simulink model "baseline_auto_parcel_loading_process"  (R2026a)
settings: Solver=VariableStepAuto  StopTime=500  MaxStep=0.05
libraries: sim3dlib x36
(part 5 of 5)

== matlab function baseline_auto_parcel_loading_process/MultiFloorUnloadPrepositionFunction ==
  data: mission_phase input size=[1 1]; unload_floor1_conv_cmd output size=[1 1]; vehicle_stopped input size=[1 1]; delivery_arrived input; target_index_f1 input size=[1 1]; found_f1 input size=[1 1]; target_id_f1 input size=[1 1]; target_index_f2 input size=[1 1]; found_f2 input size=[1 1]; target_id_f2 input size=[1 1]; target_index_f3 input size=[1 1]; found_f3 input size=[1 1]; target_id_f3 input size=[1 1]; unload_floor2_conv_cmd output size=[1 1]; unload_floor3_conv_cmd output size=[1 1]; sensor_count_f1 output size=[1 1]; sensor_count_f2 output size=[1 1]; sensor_count_f3 output size=[1 1]; target_on_belt4_f1 output size=[1 1]; target_on_belt4_f2 output size=[1 1]; target_on_belt4_f3 output size=[1 1]; preposition_active_f1 output size=[1 1]; preposition_active_f2 output size=[1 1]; preposition_active_f3 output size=[1 1]; unload_state_id_for_preposition input size=[1 1]; visual_shift_f1 output size=[1 1]; visual_shift_f2 output size=[1 1]; visual_shift_f3 output size=[1 1]
function [unload_floor1_conv_cmd, unload_floor2_conv_cmd, unload_floor3_conv_cmd, ...
          sensor_count_f1, sensor_count_f2, sensor_count_f3, ...
          target_on_belt4_f1, target_on_belt4_f2, target_on_belt4_f3, ...
          preposition_active_f1, preposition_active_f2, preposition_active_f3, ...
          visual_shift_f1, visual_shift_f2, visual_shift_f3] = ...
          MultiFloorUnloadPrepositionFunction( ...
          mission_phase, vehicle_stopped, delivery_arrived, ...
          target_index_f1, found_f1, target_id_f1, ...
          target_index_f2, found_f2, target_id_f2, ...
          target_index_f3, found_f3, target_id_f3, ...
          unload_state_id_for_preposition)
% MultiFloorUnloadPrepositionFunction
%
% 목적:
% - 배송 중 정차 시간에 각 층 컨베이어를 독립적으로 순환시켜
%   각 층의 하차 대상 1개씩을 Belt4 상단/플랫폼 앞 하차공간으로 미리 이동시킨다.
%
% 추가 목적:
% - 같은 층에 하차 대상이 여러 개 있을 때,
%   첫 번째 하차 후 다음 대상도 다시 하차공간으로 준비할 수 있게 한다.
%
% 이번 추가:
% - visual_shift_f1/f2/f3 출력
% - sensor_count는 정수 칸 이동량
% - visual_shift는 정수 칸 이동량 + 현재 카운트 사이의 진행률
%
% 핵심 규칙:
% - mission_phase == 1 일 때만 하차 준비 가능
% - vehicle_stopped == 1 일 때만 하차 준비 가능
% - 배송 중(delivery_arrived == 0)에는 정차 중이면 준비 가능
% - 배달 장소 도착 후(delivery_arrived == 1)에는 UnloadController가 IDLE일 때만 준비 가능
% - 실제 하차 중(unload_state_id 1~7)에는 준비 컨베이어 정지
% - 각 층 sensor_count는 독립적으로 관리
% - queue 자체는 회전시키지 않고, 표시용 sensor_count/visual_shift만 증가시킴
%
% 중요:
% - target_index = 1 이라고 해서 즉시 하차공간에 있다고 보지 않는다.
% - 실제 시스템의 카운팅은 "첫 번째 택배 통과 = count 1"이다.
% - 따라서 필요한 count는 target_index - 1 이 아니라 target_index 이다.

persistent count_f1 count_f2 count_f3
persistent step_f1 step_f2 step_f3
persistent done_f1 done_f2 done_f3
persistent prev_target_id_f1 prev_target_id_f2 prev_target_id_f3

if isempty(count_f1)
    count_f1 = 0;
    count_f2 = 0;
    count_f3 = 0;

    step_f1 = 0;
    step_f2 = 0;
    step_f3 = 0;

    done_f1 = 0;
    done_f2 = 0;
    done_f3 = 0;

    prev_target_id_f1 = 0;
    prev_target_id_f2 = 0;
    prev_target_id_f3 = 0;
end

% =========================
% 조정 파라미터
% =========================
% Sample time = 0.05 기준
% COUNT_INTERVAL = 20이면 약 1초마다 sensor_count가 1 증가
COUNT_INTERVAL = 60;

% =========================
% 기본 출력
% =========================
unload_floor1_conv_cmd = 0;
unload_floor2_conv_cmd = 0;
unload_floor3_conv_cmd = 0;

target_on_belt4_f1 = 0;
target_on_belt4_f2 = 0;
target_on_belt4_f3 = 0;

preposition_active_f1 = 0;
preposition_active_f2 = 0;
preposition_active_f3 = 0;

% =========================
% target 변경 감지 및 층별 카운터 리셋
% =========================
if target_id_f1 ~= prev_target_id_f1
    count_f1 = 0;
    step_f1 = 0;
    done_f1 = 0;
    prev_target_id_f1 = target_id_f1;
end

if target_id_f2 ~= prev_target_id_f2
    count_f2 = 0;
    step_f2 = 0;
    done_f2 = 0;
    prev_target_id_f2 = target_id_f2;
end

if target_id_f3 ~= prev_target_id_f3
    count_f3 = 0;
    step_f3 = 0;
    done_f3 = 0;
    prev_target_id_f3 = target_id_f3;
end

% target이 없으면 해당 층 준비 상태 리셋
if found_f1 < 0.5 || target_id_f1 <= 0
    count_f1 = 0;
    step_f1 = 0;
    done_f1 = 0;
end

if found_f2 < 0.5 || target_id_f2 <= 0
    count_f2 = 0;
    step_f2 = 0;
    done_f2 = 0;
end

if found_f3 < 0.5 || target_id_f3 <= 0
    count_f3 = 0;
    step_f3 = 0;
    done_f3 = 0;
end

% =========================
% 필요한 sensor count 계산
% =========================
need_f1 = target_index_f1;
need_f2 = target_index_f2;
need_f3 = target_index_f3;

if need_f1 < 0
    need_f1 = 0;
end

if need_f2 < 0
    need_f2 = 0;
end

if need_f3 < 0
    need_f3 = 0;
end

if found_f1 < 0.5 || target_id_f1 <= 0
    need_f1 = 0;
end

if found_f2 < 0.5 || target_id_f2 <= 0
    need_f2 = 0;
end

if found_f3 < 0.5 || target_id_f3 <= 0
    need_f3 = 0;
end

% =========================
% 준비 완료 판정
% =========================
if found_f1 > 0.5 && target_id_f1 > 0
    if count_f1 >= need_f1
        done_f1 = 1;
    end
end

if found_f2 > 0.5 && target_id_f2 > 0
    if count_f2 >= need_f2
        done_f2 = 1;
    end
end

if found_f3 > 0.5 && target_id_f3 > 0
    if count_f3 >= need_f3
        done_f3 = 1;
    end
end

% =========================
% 하차 준비 허용 조건
% =========================
% 배송 중:
%   delivery_arrived = 0
%   vehicle_stopped = 1
%   → 준비 가능
%
% 배달 장소 도착 후:
%   delivery_arrived = 1
%   unload_state_id_for_preposition = 0
%   → 실제 하차 중이 아닐 때만 다음 대상 준비 가능
%
% 실제 하차 중:
%   unload_state_id_for_preposition ~= 0
%   → 준비 컨베이어 정지
prep_allowed = 0;

if mission_phase == 1 && vehicle_stopped > 0.5

    if delivery_arrived <= 0.5
        prep_allowed = 1;

    else
        if unload_state_id_for_preposition <= 0.5
            prep_allowed = 1;
        else
            prep_allowed = 0;
        end
    end

end

% =========================
% 1층 준비
% =========================
if found_f1 > 0.5 && target_id_f1 > 0 && done_f1 < 0.5
    if prep_allowed > 0.5
        preposition_active_f1 = 1;
        unload_floor1_conv_cmd = 1;

        step_f1 = step_f1 + 1;

        if step_f1 >= COUNT_INTERVAL
            step_f1 = 0;
            count_f1 = count_f1 + 1;
        end
    end
end

% =========================
% 2층 준비
% =========================
if found_f2 > 0.5 && target_id_f2 > 0 && done_f2 < 0.5
    if prep_allowed > 0.5
        preposition_active_f2 = 1;
        unload_floor2_conv_cmd = 1;

        step_f2 = step_f2 + 1;

        if step_f2 >= COUNT_INTERVAL
            step_f2 = 0;
            count_f2 = count_f2 + 1;
        end
    end
end

% =========================
% 3층 준비
% =========================
if found_f3 > 0.5 && target_id_f3 > 0 && done_f3 < 0.5
    if prep_allowed > 0.5
        preposition_active_f3 = 1;
        unload_floor3_conv_cmd = 1;

        step_f3 = step_f3 + 1;

        if step_f3 >= COUNT_INTERVAL
            step_f3 = 0;
            count_f3 = count_f3 + 1;
        end
    end
end

% =========================
% 준비 완료 재판정
% =========================
if found_f1 > 0.5 && target_id_f1 > 0
    if count_f1 >= need_f1
        done_f1 = 1;
    end
end

if found_f2 > 0.5 && target_id_f2 > 0
    if count_f2 >= need_f2
        done_f2 = 1;
    end
end

if found_f3 > 0.5 && target_id_f3 > 0
    if count_f3 >= need_f3
        done_f3 = 1;
    end
end

% =========================
% 출력
% =========================
sensor_count_f1 = count_f1;
sensor_count_f2 = count_f2;
sensor_count_f3 = count_f3;

if done_f1 > 0.5 && found_f1 > 0.5 && target_id_f1 > 0
    target_on_belt4_f1 = 1;
else
    target_on_belt4_f1 = 0;
end

if done_f2 > 0.5 && found_f2 > 0.5 && target_id_f2 > 0
    target_on_belt4_f2 = 1;
else
    target_on_belt4_f2 = 0;
end

if done_f3 > 0.5 && found_f3 > 0.5 && target_id_f3 > 0
    target_on_belt4_f3 = 1;
else
    target_on_belt4_f3 = 0;
end

% =========================
% 연속 이동 시각화용 출력
% =========================
% done 상태가 아니고, 실제로 준비 active 중일 때는
% count + step/COUNT_INTERVAL 값을 내보낸다.
%
% done 상태에서는 step이 남아 있어도 정수 count 위치로 고정한다.
if done_f1 < 0.5 && preposition_active_f1 > 0.5
    visual_shift_f1 = count_f1 + step_f1 / COUNT_INTERVAL;
else
    visual_shift_f1 = count_f1;
end

if done_f2 < 0.5 && preposition_active_f2 > 0.5
    visual_shift_f2 = count_f2 + step_f2 / COUNT_INTERVAL;
else
    visual_shift_f2 = count_f2;
end

if done_f3 < 0.5 && preposition_active_f3 > 0.5
    visual_shift_f3 = count_f3 + step_f3 / COUNT_INTERVAL;
else
    visual_shift_f3 = count_f3;
end

end

== matlab function baseline_auto_parcel_loading_process/CurrentUnloadReadySelector ==
  data: target_unload_floor input; current_target_on_belt4 output; target_on_belt4_f1 input; target_on_belt4_f2 input; target_on_belt4_f3 input
function current_target_on_belt4 = CurrentUnloadReadySelector(target_unload_floor, target_on_belt4_f1, target_on_belt4_f2, target_on_belt4_f3)
% CurrentUnloadReadySelector
%
% 현재 실제로 하차할 target이 어느 층에 있는지 보고,
% 그 층의 준비 완료 신호만 UnloadController로 전달한다.

current_target_on_belt4 = 0;

if target_unload_floor == 1
    current_target_on_belt4 = target_on_belt4_f1;

elseif target_unload_floor == 2
    current_target_on_belt4 = target_on_belt4_f2;

elseif target_unload_floor == 3
    current_target_on_belt4 = target_on_belt4_f3;

else
    current_target_on_belt4 = 0;
end

end

== matlab function baseline_auto_parcel_loading_process/Floor2VisualStateFunction ==
  data: floor2_queue input; floor2_visual_id output size=[6 1]; visual_shift_f2 input; target_id_f2 input; target_on_belt4_f2 input; current_unload_id input; package_on_platform_from_floor input; unload_done input; floor2_visual_path output size=[6 1]; floor2_visual_count output size=[1 1]; belt4_reverse_cmd input; belt4_restore_cmd input; belt4_reverse_progress output size=[1 1]; belt4_reverse_phase output size=[1 1]
function [floor2_visual_id, floor2_visual_path, floor2_visual_count, belt4_reverse_progress, belt4_reverse_phase] = ...
    Floor2VisualStateFunction(floor2_queue, visual_shift_f2, target_id_f2, target_on_belt4_f2, ...
                              current_unload_id, package_on_platform_from_floor, unload_done, ...
                              belt4_reverse_cmd, belt4_restore_cmd)
% Floor2VisualStateFunction
%
% 목적:
% - 2층 박스들의 시각적 벨트 위치를 따로 저장한다.
% - floor2_queue는 논리 queue이므로 하차 완료 시 압축될 수 있다.
% - visual state는 실제 벨트 위 위치를 유지한다.
%
% 중요:
% - queue에 없다는 이유로 visual state에서 제거하지 않는다.
% - 실제 하차 완료된 carried_id만 unload_done 상승엣지에서 삭제한다.
% - Belt4 reverse/restore는 2층 하차 대상일 때만 동작한다.
% - reverse_progress는 persistent로 유지되어야 하며 매 스텝 0으로 초기화하면 안 된다.

MAX_VISUAL = 6;
QUEUE_MAX = 50;

persistent ids
persistent paths
persistent prev_shift
persistent initialized
persistent carried_id
persistent prev_unload_done

persistent reverse_progress
persistent reverse_phase
persistent prev_reverse_cmd
persistent prev_restore_cmd

if isempty(initialized)
    ids = zeros(MAX_VISUAL, 1);
    paths = zeros(MAX_VISUAL, 1);
    prev_shift = 0;
    initialized = 1;

    carried_id = 0;
    prev_unload_done = 0;

    reverse_progress = 0;
    reverse_phase = 0;
    prev_reverse_cmd = 0;
    prev_restore_cmd = 0;
end

% =========================
% 기본 출력 초기화
% =========================
floor2_visual_id = zeros(MAX_VISUAL, 1);
floor2_visual_path = zeros(MAX_VISUAL, 1);
floor2_visual_count = 0;
belt4_reverse_progress = reverse_progress;
belt4_reverse_phase = reverse_phase;

% =========================
% 1. queue에 새로 생긴 package를 visual state에 등록
% =========================
for q = 1:QUEUE_MAX
    pkg_id = floor2_queue(q);

    if pkg_id > 0
        exists = 0;

        for k = 1:MAX_VISUAL
            if ids(k) == pkg_id
                exists = 1;
            end
        end

        if exists < 0.5
            free_idx = 0;

            for k = 1:MAX_VISUAL
                if ids(k) <= 0 && free_idx == 0
                    free_idx = k;
                end
            end

            if free_idx > 0
                ids(free_idx) = pkg_id;
                paths(free_idx) = q;
            end
        end
    end
end

% =========================
% 2. queue에서 사라진 package 제거 금지
% =========================
% floor2_queue는 논리 queue이므로 하차 완료 후 압축될 수 있다.
% visual state는 실제 벨트 위 위치를 표현하므로,
% queue에 없다는 이유만으로 삭제하지 않는다.

% =========================
% 3. 플랫폼 위에 올라간 package ID 기억
% =========================
if package_on_platform_from_floor > 0.5 && current_unload_id > 0
    carried_id = current_unload_id;
end

% =========================
% 4. unload_done 상승엣지에서 carried_id 제거
% =========================
unload_done_rise = 0;

if unload_done > 0.5 && prev_unload_done <= 0.5
    unload_done_rise = 1;
end

if unload_done_rise > 0.5 && carried_id > 0
    for k = 1:MAX_VISUAL
        if ids(k) == carried_id
            ids(k) = 0;
            paths(k) = 0;
        end
    end

    carried_id = 0;
end

prev_unload_done = unload_done;

% =========================
% 5. visual_shift 변화량으로 모든 박스 이동
% =========================
delta = visual_shift_f2 - prev_shift;

% target 전환 시 visual_shift가 리셋되면 뒤로 돌아가지 않게 한다.
if delta < 0
    delta = 0;
    prev_shift = visual_shift_f2;
end

% 너무 큰 점프 방지
if delta > 1
    delta = 1;
end

% target이 하차공간을 지나 과도하게 이동하지 않도록 제한
if delta > 0
    target_path = 999;

    if target_id_f2 > 0
        for k = 1:MAX_VISUAL
            if ids(k) == target_id_f2
                target_path = paths(k);
            end
        end
    end

    if target_path <= 0
        delta = 0;
    elseif delta > target_path
        delta = target_path;
    end
end

% 준비 완료 상태에서는 더 이상 하차공간 방향 순환 이동을 하지 않음
if target_on_belt4_f2 > 0.5
    delta = 0;
end

if delta > 0
    for k = 1:MAX_VISUAL
        if ids(k) > 0
            paths(k) = paths(k) - delta;
        end
    end
end

if visual_shift_f2 >= prev_shift
    prev_shift = visual_shift_f2;
end

% =========================
% 6. Belt4 reverse/restore 동작
% =========================
% reverse_progress = 0 : Belt4 원위치
% reverse_progress = 1 : 하차 대상 박스가 플랫폼 위로 충분히 밀린 상태
%
% 중요:
% - belt4_reverse_cmd는 전 층 공통 신호일 수 있으므로,
%   2층 하차 대상일 때만 local_reverse_cmd를 허용한다.
% - restore는 reverse_progress가 실제로 0보다 클 때만 허용한다.
% - reverse_cmd가 짧게 들어와도 reverse_phase가 latch되어 1까지 진행된다.

Ts_reverse = 0.05;
reverse_speed = 0.30;       % 0 -> 1까지 약 3.3초
reverse_step = reverse_speed * Ts_reverse;

is_current_floor2_unload = 0;

if target_id_f2 > 0 && current_unload_id > 0
    if target_id_f2 == current_unload_id
        is_current_floor2_unload = 1;
    end
end

local_reverse_cmd = 0;
local_restore_cmd = 0;

% 2층 대상이 하차공간에 있고, 현재 하차 대상도 2층 target일 때만 reverse 시작
if belt4_reverse_cmd > 0.5 && is_current_floor2_unload > 0.5 && target_on_belt4_f2 > 0.5
    local_reverse_cmd = 1;
end

% reverse_progress가 실제로 진행된 층만 restore 허용
if belt4_restore_cmd > 0.5 && reverse_progress > 0
    local_restore_cmd = 1;
end

reverse_cmd_rise = 0;
restore_cmd_rise = 0;

if local_reverse_cmd > 0.5 && prev_reverse_cmd <= 0.5
    reverse_cmd_rise = 1;
end

if local_restore_cmd > 0.5 && prev_restore_cmd <= 0.5
    restore_cmd_rise = 1;
end

prev_reverse_cmd = local_reverse_cmd;
prev_restore_cmd = local_restore_cmd;

if reverse_cmd_rise > 0.5
    reverse_phase = 1;
end

if restore_cmd_rise > 0.5
    reverse_phase = 2;
end

if reverse_phase == 1

    reverse_progress = reverse_progress + reverse_step;

    if reverse_progress >= 1
        reverse_progress = 1;
        reverse_phase = 0;
    end

elseif reverse_phase == 2

    reverse_progress = reverse_progress - reverse_step;

    if reverse_progress <= 0
        reverse_progress = 0;
        reverse_phase = 0;
    end

end

belt4_reverse_progress = reverse_progress;
belt4_reverse_phase = reverse_phase;

% =========================
% 7. 출력 정리
% =========================
count = 0;

% Belt4 위 다른 박스들의 역회전 표시 이동량
% 너무 크게 주면 path가 0을 넘어 Belt3 위치로 넘어가 보인다.
% 하차 대상 박스는 F2 makePkg에서 별도로 플랫폼까지 크게 이동시키므로,
% 여기서는 Belt4 위 다른 박스들의 '같이 밀림'만 작게 표현한다.
NON_TARGET_REVERSE_TRAVEL = 1.5;

for k = 1:MAX_VISUAL
    floor2_visual_id(k) = ids(k);

    display_path = paths(k);

    if reverse_progress > 0
        if ids(k) > 0 && paths(k) <= 0

            % 현재 하차 대상은 F2 makePkg에서 handoff -> platform으로 별도 표시한다.
            % 여기서는 하차 대상이 아닌 Belt4 위 박스만 살짝 밀었다가 복귀시킨다.
            if ids(k) ~= current_unload_id
                display_path = paths(k) + reverse_progress * NON_TARGET_REVERSE_TRAVEL;

                % 절대 하차공간/벨트3 쪽으로 넘어가지 않게 제한한다.
                % path > 0이 되면 getIntegerPose에서 Belt3 슬롯으로 해석되기 때문.
                if display_path > -0.05
                    display_path = -0.05;
                end
            end
        end
    end

    floor2_visual_path(k) = display_path;

    if ids(k) > 0
        count = count + 1;
    end
end

floor2_visual_count = count;

end

== matlab function baseline_auto_parcel_loading_process/Floor1VisualStateFunction ==
  data: floor1_queue input; floor1_visual_id output size=[5 1]; visual_shift_f1 input; target_id_f1 input; target_on_belt4_f1 input; current_unload_id input; package_on_platform_from_floor input; unload_done input; floor1_visual_path output size=[5 1]; floor1_visual_count output size=[1 1]; belt4_reverse_cmd input; belt4_restore_cmd input; belt4_reverse_progress output size=[1 1]; belt4_reverse_phase output size=[1 1]
function [floor1_visual_id, floor1_visual_path, floor1_visual_count, belt4_reverse_progress, belt4_reverse_phase] = ...
    Floor1VisualStateFunction(floor1_queue, visual_shift_f1, target_id_f1, target_on_belt4_f1, ...
                              current_unload_id, package_on_platform_from_floor, unload_done, ...
                              belt4_reverse_cmd, belt4_restore_cmd)
% Floor1VisualStateFunction
%
% 목적:
% - 1층 박스들의 시각적 벨트 위치를 따로 저장한다.
% - floor1_queue는 논리 queue이므로 하차 완료 시 압축될 수 있다.
% - visual state는 실제 벨트 위 위치를 유지한다.
%
% 핵심:
% - queue에 없다는 이유로 visual state에서 제거하지 않는다.
% - 실제 하차 완료된 carried_id만 unload_done 상승엣지에서 삭제한다.
% - Belt4 reverse/restore는 1층 하차 대상일 때만 동작한다.
% - reverse_progress는 persistent로 유지되어야 하며 매 스텝 초기화하면 안 된다.

MAX_VISUAL = 5;
QUEUE_MAX = 50;

persistent ids
persistent paths
persistent prev_shift
persistent initialized
persistent carried_id
persistent prev_unload_done

persistent reverse_progress
persistent reverse_phase
persistent prev_reverse_cmd
persistent prev_restore_cmd

if isempty(initialized)
    ids = zeros(MAX_VISUAL, 1);
    paths = zeros(MAX_VISUAL, 1);
    prev_shift = 0;
    initialized = 1;

    carried_id = 0;
    prev_unload_done = 0;

    reverse_progress = 0;
    reverse_phase = 0;
    prev_reverse_cmd = 0;
    prev_restore_cmd = 0;
end

% =========================
% 기본 출력 초기화
% =========================
floor1_visual_id = zeros(MAX_VISUAL, 1);
floor1_visual_path = zeros(MAX_VISUAL, 1);
floor1_visual_count = 0;

belt4_reverse_progress = reverse_progress;
belt4_reverse_phase = reverse_phase;

% =========================
% 1. queue에 새로 생긴 package를 visual state에 등록
% =========================
for q = 1:QUEUE_MAX
    pkg_id = floor1_queue(q);

    if pkg_id > 0
        exists = 0;

        for k = 1:MAX_VISUAL
            if ids(k) == pkg_id
                exists = 1;
            end
        end

        if exists < 0.5
            free_idx = 0;

            for k = 1:MAX_VISUAL
                if ids(k) <= 0 && free_idx == 0
                    free_idx = k;
                end
            end

            if free_idx > 0
                ids(free_idx) = pkg_id;
                paths(free_idx) = q;
            end
        end
    end
end

% =========================
% 2. queue에서 사라진 package 제거 금지
% =========================
% floor1_queue는 논리 queue이므로 하차 완료 후 압축될 수 있다.
% visual state는 실제 벨트 위 위치를 표현하므로,
% queue에 없다는 이유만으로 삭제하지 않는다.

% =========================
% 3. 플랫폼 위에 올라간 package ID 기억
% =========================
if package_on_platform_from_floor > 0.5 && current_unload_id > 0
    carried_id = current_unload_id;
end

% =========================
% 4. unload_done 상승엣지에서 carried_id 제거
% =========================
unload_done_rise = 0;

if unload_done > 0.5 && prev_unload_done <= 0.5
    unload_done_rise = 1;
end

if unload_done_rise > 0.5 && carried_id > 0
    for k = 1:MAX_VISUAL
        if ids(k) == carried_id
            ids(k) = 0;
            paths(k) = 0;
        end
    end

    carried_id = 0;
end

prev_unload_done = unload_done;

% =========================
% 5. visual_shift 변화량으로 모든 박스 이동
% =========================
delta = visual_shift_f1 - prev_shift;

% target 전환 시 visual_shift가 리셋되면 뒤로 돌아가지 않게 한다.
if delta < 0
    delta = 0;
    prev_shift = visual_shift_f1;
end

% 너무 큰 점프 방지
if delta > 1
    delta = 1;
end

% target이 하차공간을 지나 과도하게 이동하지 않도록 제한
if delta > 0
    target_path = 999;

    if target_id_f1 > 0
        for k = 1:MAX_VISUAL
            if ids(k) == target_id_f1
                target_path = paths(k);
            end
        end
    end

    if target_path <= 0
        delta = 0;
    elseif delta > target_path
        delta = target_path;
    end
end

% 준비 완료 상태에서는 더 이상 하차공간 방향 순환 이동을 하지 않음
if target_on_belt4_f1 > 0.5
    delta = 0;
end

if delta > 0
    for k = 1:MAX_VISUAL
        if ids(k) > 0
            paths(k) = paths(k) - delta;
        end
    end
end

if visual_shift_f1 >= prev_shift
    prev_shift = visual_shift_f1;
end

% =========================
% 6. Belt4 reverse/restore 동작
% =========================
% reverse_progress = 0 : Belt4 원위치
% reverse_progress = 1 : 하차 대상 박스가 플랫폼 위로 충분히 밀린 상태
%
% 중요:
% - belt4_reverse_cmd는 전 층 공통 신호일 수 있으므로,
%   1층 하차 대상일 때만 local_reverse_cmd를 허용한다.
% - restore는 reverse_progress가 실제로 0보다 클 때만 허용한다.
% - reverse_cmd가 짧게 들어와도 reverse_phase가 latch되어 1까지 진행된다.

Ts_reverse = 0.05;
reverse_speed = 0.30;
reverse_step = reverse_speed * Ts_reverse;

is_current_floor1_unload = 0;

if target_id_f1 > 0 && current_unload_id > 0
    if target_id_f1 == current_unload_id
        is_current_floor1_unload = 1;
    end
end

local_reverse_cmd = 0;
local_restore_cmd = 0;

% 1층 대상이 하차공간에 있고, 현재 하차 대상도 1층 target일 때만 reverse 시작
if belt4_reverse_cmd > 0.5 && is_current_floor1_unload > 0.5 && target_on_belt4_f1 > 0.5
    local_reverse_cmd = 1;
end

% reverse_progress가 실제로 진행된 층만 restore 허용
if belt4_restore_cmd > 0.5 && reverse_progress > 0
    local_restore_cmd = 1;
end

reverse_cmd_rise = 0;
restore_cmd_rise = 0;

if local_reverse_cmd > 0.5 && prev_reverse_cmd <= 0.5
    reverse_cmd_rise = 1;
end

if local_restore_cmd > 0.5 && prev_restore_cmd <= 0.5
    restore_cmd_rise = 1;
end

prev_reverse_cmd = local_reverse_cmd;
prev_restore_cmd = local_restore_cmd;

if reverse_cmd_rise > 0.5
    reverse_phase = 1;
end

if restore_cmd_rise > 0.5
    reverse_phase = 2;
end

if reverse_phase == 1

    reverse_progress = reverse_progress + reverse_step;

    if reverse_progress >= 1
        reverse_progress = 1;
        reverse_phase = 0;
    end

elseif reverse_phase == 2

    reverse_progress = reverse_progress - reverse_step;

    if reverse_progress <= 0
        reverse_progress = 0;
        reverse_phase = 0;
    end

end

belt4_reverse_progress = reverse_progress;
belt4_reverse_phase = reverse_phase;

% =========================
% 7. 출력 정리
% =========================
count = 0;

% 하차 대상이 아닌 Belt4 위 박스들의 역회전 표시 이동량
% 너무 크게 주면 path가 0을 넘어 Belt3 위치로 넘어가 보인다.
NON_TARGET_REVERSE_TRAVEL = 1.5;

for k = 1:MAX_VISUAL
    floor1_visual_id(k) = ids(k);

    display_path = paths(k);

    if reverse_progress > 0
        if ids(k) > 0 && paths(k) <= 0

            % 현재 하차 대상은 F1 makePkg에서 handoff -> platform으로 별도 표시한다.
            % 여기서는 하차 대상이 아닌 Belt4 위 박스만 살짝 밀었다가 복귀시킨다.
            if ids(k) ~= current_unload_id
                display_path = paths(k) + reverse_progress * NON_TARGET_REVERSE_TRAVEL;

                % path > 0이 되면 Belt3 슬롯으로 해석되므로 방지한다.
                if display_path > -0.05
                    display_path = -0.05;
                end
            end
        end
    end

    floor1_visual_path(k) = display_path;

    if ids(k) > 0
        count = count + 1;
    end
end

floor1_visual_count = count;

end

== matlab function baseline_auto_parcel_loading_process/TargetFloorSelector ==
  data: box_insert_length input; target_floor output; floor1_used_length input; floor2_used_length input; floor3_used_length input; floor_capacity_length input; storage_available output; floor1_remaining_length output; floor2_remaining_length output; floor3_remaining_length output
function [target_floor, storage_available, floor1_remaining_length, floor2_remaining_length, floor3_remaining_length] = TargetFloorSelector(box_insert_length, floor1_used_length, floor2_used_length, floor3_used_length, floor_capacity_length)
% TargetFloorSelector
% 각 층의 남은 적재 길이를 계산하고,
% box_insert_length가 들어갈 수 있는 층 중 best-fit 방식으로 목표층을 선택한다.
%
% best-fit:
% 들어갈 수 있는 층 중에서 넣고 난 뒤 남는 길이가 가장 작은 층 선택

floor1_remaining_length = floor_capacity_length - floor1_used_length;
floor2_remaining_length = floor_capacity_length - floor2_used_length;
floor3_remaining_length = floor_capacity_length - floor3_used_length;

storage_available = 0;
target_floor = 0;

best_leftover = 1.0e9;

% 1층 검사
if box_insert_length <= floor1_remaining_length
    leftover = floor1_remaining_length - box_insert_length;
    if leftover < best_leftover
        best_leftover = leftover;
        target_floor = 1;
        storage_available = 1;
    end
end

% 2층 검사
if box_insert_length <= floor2_remaining_length
    leftover = floor2_remaining_length - box_insert_length;
    if leftover < best_leftover
        best_leftover = leftover;
        target_floor = 2;
        storage_available = 1;
    end
end

% 3층 검사
if box_insert_length <= floor3_remaining_length
    leftover = floor3_remaining_length - box_insert_length;
    if leftover < best_leftover
        best_leftover = leftover;
        target_floor = 3;
        storage_available = 1;
    end
end

% 어디에도 못 넣으면 target_floor = 0
if storage_available == 0
    target_floor = 0;
end
